simulink model "UNIFIER"  (R2023b)
settings: Solver=ode1  StartTime=0.0  StopTime=60  FixedStep=1/500  RelTol=1e-3
values from neighbouring files (symbols this model uses):
  b = 20.11467    [UNIFIER_LOAD.m]
  c = 1.43676    [UNIFIER_LOAD.m]
  DEP_INTEG_IC = 117.49388    [UNIFIER_LOAD.m]
  Euler0 = [3.43106170068520e-06, 0.0515008506277664, -2.79252663434261]    [UNIFIER_LOAD.m]
  ground_alt = 0    [UNIFIER_LOAD.m]
  h_ref_for_xplane = 0    [UNIFIER_LOAD.m]
  m = 7057    [UNIFIER_LOAD.m]
  omegab0 = [0,0,0]    [UNIFIER_LOAD.m]
  S = 29.98388    [UNIFIER_LOAD.m]
  sensor_delay_steps = 5    [UNIFIER_LOAD.m]
  u1_0 = [2.1112539e-05, -2.1112539e-05, -0.085004635, -0.084972650, 0.19720161, 0.19720161]    [UNIFIER_LOAD.m]
  u2_0 = ones(1,12) .* 0.4252    [UNIFIER_LOAD.m]
  u3_0 = 0.089689    [UNIFIER_LOAD.m]
  u4_0 = 0    [UNIFIER_LOAD.m]
  Vb0 = [52.6789583501891, 0, 2.71559652634250]    [UNIFIER_LOAD.m]
  vtail_dist_to_wing = 7.8070    (= 7.807)    [UNIFIER_LOAD.m]
  vtail_nodes = [dp_VTAIL.Xs_LE;     dp_VTAIL.Ys_LE;     dp_VTAIL.Zs_LE]    [UNIFIER_LOAD.m]
  wing_nodes = [fliplr(dp_WING_tip.LE_Xs),fliplr(dp_WING_root.LE_Xs),dp_WING_root.LE_Xs,dp_WING_tip.LE_Xs;     fliplr(-dp_WING_tip.LE_Ys),fliplr(-dp_WING_root.LE_Ys),dp_WING_root.LE_Ys,dp_WING_tip.LE_Ys;     fliplr(dp_WING_tip.LE_Zs),fliplr(dp_WING_root.LE_Zs),dp_WING_root.LE_Zs,dp_WING_tip.LE_Zs]    [UNIFIER_LOAD.m]
  Xe0 = [0,0,-1100]    [UNIFIER_LOAD.m]
  xyz_cg = [-8.09,0,-0.2]    [UNIFIER_LOAD.m]
  xyz_DEP = [ -6.9629998	-6.9210000	-6.8660002	-6.8099999	-6.7540002	-6.6999998	-6.6999998	-6.7540002	-6.8099999	-6.8660002	-6.9210000	-6.9629998 ... (first row only)    [UNIFIER_LOAD.m]
undefined symbols (not defined in the file or in its folder): dp_DEP, dp_FUSE_FIN, dp_HTU, dp_VTAIL, dp_VTAIL_INDUCED, dp_WING_root, dp_WING_tip, Earth, F, fcc, MIL, WGS84
libraries: aerolibactuator x16, dspnetwork x15, sharedutil x14, simulink_extras x13, sharedtransform x7, aerolibtransform2 x5, simulink x5, aerolibwind2 x4, matrix_library x1, shared6dof x1, aerolibatmos2 x1, slpidlib x1
(part 1 of 4)
settings Model: SimulationMode=rapid-accelerator  PauseTimes=1.5  Creator=johannes  LastModifiedBy=johannes
settings DebuggingCC: ParameterPrecisionLossMsg=none  UnconnectedInputMsg=warning  UnconnectedOutputMsg=warning  UnconnectedLineMsg=warning  UnitsInconsistencyMsg=none  AllowAutomaticUnitConversions=off
settings ModelReferenceCC: EnableRefExpFcnMdlSchedulingChecks=on
settings RTWCC: DLArmComputeVersion=19.05

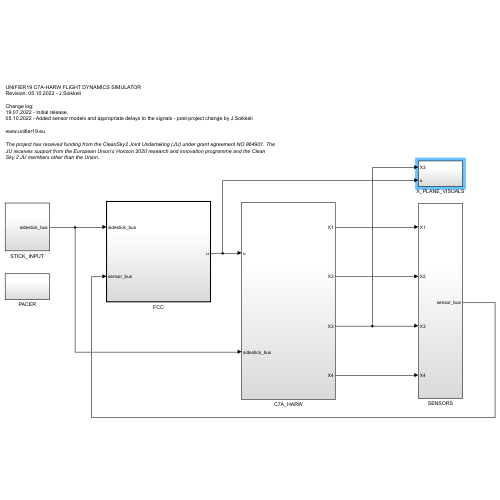
[thumbnail: Simulink's stored preview of the top-level diagram]
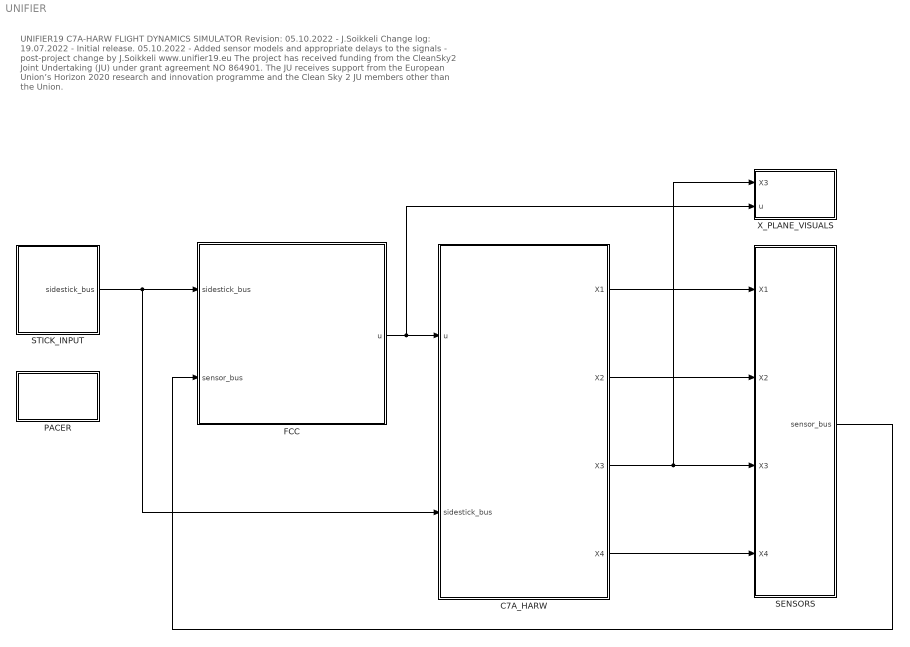
== system UNIFIER ==
  note: UNIFIER19 C7A-HARW FLIGHT DYNAMICS SIMULATOR
      | Revision: 05.10.2022 - J.Soikkeli
      |
      | Change log:
      | 19.07.2022 - Initial release.
      | 05.10.2022 - Added sensor models and appropriate delays to the signals - post-project change by J.Soikkeli
      |
      | www.unifier19.eu
      |
      | The project has received funding from the CleanSky2 Joint Undertaking (JU) under grant agreement NO 864901. The JU receives support from the European Union’s Horizon 2020 research and innovation programme and the Clean Sky 2 JU members other than the Union.
  C7A_HARW : Subsystem
  FCC : Subsystem  TreatAsAtomicUnit=on  SystemSampleTime=fcc.dt
  PACER : Subsystem
  SENSORS : Subsystem
  STICK_INPUT : Subsystem
  X_PLANE_VISUALS : Subsystem
  wires:
  C7A_HARW/3(X3) -> SENSORS/3(X3), X_PLANE_VISUALS/1(X3)
  FCC/1(u) -> X_PLANE_VISUALS/2(u), C7A_HARW/1(u)
  C7A_HARW/1(X1) -> SENSORS/1(X1)
  C7A_HARW/2(X2) -> SENSORS/2(X2)
  C7A_HARW/4(X4) -> SENSORS/4(X4)
  SENSORS/1(sensor_bus) -> FCC/2(sensor_bus)
  STICK_INPUT/1(sidestick_bus) -> C7A_HARW/2(sidestick_bus), FCC/1(sidestick_bus)

== system UNIFIER/C7A_HARW ==
  u : Inport
  sidestick_bus : Inport  Port=2
  Actuator processing and transport delay 10 ms : Delay  DelayLength=5  InitialCondition=repmat([u1_0,u2_0,u3_0,u4_0]',1,5)
  Aero : Subsystem
  Bus Selector : BusSelector  OutputSignals=V_rw_tas,omega_rw,V_rw_mag_tas,beta,alpha,rho
  Cast{1,6..12} (8 alike) : DataTypeConversion  OutDataTypeStr=single  SaturateOnIntegerOverflow=off  RndMeth=Floor
  Demux : Demux  Outputs=[6,12,1,1]
  EOMandEnviroment1 : Subsystem
  FCC frame delay 10 ms (assumed 100Hz FCC) : Delay  DelayLength=5  InitialCondition=repmat([u1_0,u2_0,u3_0,u4_0]',1,5)
  Scopes : Subsystem
  Subsystems : Subsystem
  Sum : Sum  Inputs=|++
  Sum1 : Sum  Inputs=|++
  X1 : Outport
  X2 : Outport  Port=2
  X3 : Outport  Port=3
  X4 : Outport  Port=4
  wires:
  Aero/2(M) -> Sum1/1
  Bus Selector/1 -> Cast7/1  "<V_rw_tas>"
  Bus Selector/6 -> Cast8/1  "<rho>"
  Bus Selector/2 -> Cast9/1  "<omega_rw>"
  Cast6/1 -> Aero/7(DEP_J)
  Subsystems/1(DEP_J) -> Cast6/1
  Subsystems/3(F) -> Sum/2
  Aero/1(F) -> Sum/1
  Sum/1 -> EOMandEnviroment1/1(F)
  Sum1/1 -> EOMandEnviroment1/2(M)
  Subsystems/4(M) -> Sum1/2
  Bus Selector/3 -> Cast10/1  "<V_rw_mag_tas>"
  Bus Selector/4 -> Cast11/1  "<beta>"
  Bus Selector/5 -> Cast12/1  "<alpha>"
  Cast7/1 -> Aero/1(V_rw_tas)
  Cast8/1 -> Aero/6(rho)
  Cast9/1 -> Aero/2(omega_rw)
  Cast10/1 -> Aero/3(V_rw_mag_tas)
  Cast11/1 -> Aero/4(beta)
  Cast12/1 -> Aero/5(alpha)
  Cast1/1 -> Aero/8(u1 (rad))
  Subsystems/2(u1_out (rad)) -> Cast1/1
  EOMandEnviroment1/1(X1) -> Scopes/1(X1), X1/1
  EOMandEnviroment1/4(X4) -> Scopes/4(X4), X4/1, Subsystems/1(X4), Bus Selector/1
  EOMandEnviroment1/2(X2) -> Subsystems/7(X2), X2/1, Scopes/2(X2)
  EOMandEnviroment1/3(X3) -> Subsystems/6(X3), X3/1, Scopes/3(X3)
  Demux/4 -> Aero/9(u4 (gear))
  sidestick_bus/1 -> Subsystems/5(sidestick_bus)
  Demux/3 -> Subsystems/4(u3 (actf))
  Demux/2 -> Subsystems/3(u2 (actf))
  Demux/1 -> Subsystems/2(u1_in (rad))
  u/1 -> FCC frame delay 10 ms (assumed 100Hz FCC)/1
  FCC frame delay 10 ms (assumed 100Hz FCC)/1 -> Actuator processing and transport delay 10 ms/1
  Actuator processing and transport delay 10 ms/1 -> Demux/1

== system UNIFIER/FCC ==
  note: As a part of the UNIFIER19 project, flight control laws (based on non-linear dynamic inversion) were developed. The litearature and findings using these control laws is available on the GIT page.
      |
      | Here we invite you to develop your version of the control laws!
  sidestick_bus : Inport
  sensor_bus : Inport  Port=2
  Bus Selector : BusSelector  OutputSignals=roll_raw,pitch_raw,yaw_raw,throttle_raw
  Constant1 : Constant  Value=u2_0
  Constant2 : Constant  Value=u3_0
  Constant3 : Constant  Value=u1_0
  Constant4 : Constant  SampleTime=-1
  Constant6 : Constant  Value=u4_0
  Manual : Subsystem
  Multiport Switch : MultiPortSwitch  Inputs=2  SaturateOnIntegerOverflow=off  InputSameDT=off
  Mux : Mux
  Terminator : Terminator
  u : Outport
  wires:
  Multiport Switch/1 -> u/1
  Constant3/1 -> Mux/1
  Constant1/1 -> Mux/2
  Constant2/1 -> Mux/3
  Mux/1 -> Multiport Switch/2
  Bus Selector/1 -> Manual/1(aileron)  "<roll_raw>"
  Bus Selector/2 -> Manual/2(elevator)  "<pitch_raw>"
  Bus Selector/3 -> Manual/3(rudder)  "<yaw_raw>"
  Bus Selector/4 -> Manual/4(throttle)  "<throttle_raw>"
  Constant4/1 -> Multiport Switch/1
  Manual/1(u) -> Multiport Switch/3
  Constant6/1 -> Mux/4
  sidestick_bus/1 -> Bus Selector/1
  sensor_bus/1 -> Terminator/1

== system UNIFIER/PACER ==
  note: Soft real time block and associated
      | s-function source codes:
      | - sfun_sleep.c
      | - sfun_getSystemClockTimeval.c
      | - sfun_output_to_console.c
      | are copyrighted
      | by Marc Compere
      | comperem@gmail.com
      | created : 28 May 2018
      | modified: 28 May 2018
  Constant1 : Constant  Value=0
  Constant2 : Constant
  Display : Display
  Manual Switch1 : ManualSwitch  CurrentSetting=0
  Mux : Mux  Inputs=3
  Output to Console : Subsystem  TreatAsAtomicUnit=on
  Subsystem : Subsystem
      settings: OpenFcn=h_fixed=0.001
      mask Display: fprintf('Double-Click to init\nstepsize variable, h_fixed')
  "pace error (s) " : Scope
  simulation time (s)1 : Clock
  soft real time subsystem : Subsystem  mask{t_sample=0.01}
      mask prompts: t_sample "Sleep function interval (s)"
  wires:
  soft real time subsystem/2(pace error (s)) -> "pace error (s) "/1, Display/1, Mux/3
  simulation time (s)1/1 -> Mux/1
  soft real time subsystem/1(t_elapsed_wall_clock (s)) -> Mux/2
  Constant1/1 -> Manual Switch1/2
  Mux/1 -> Output to Console/1(data to console)
  Constant2/1 -> Manual Switch1/1
  Manual Switch1/1 -> Output to Console/Enable

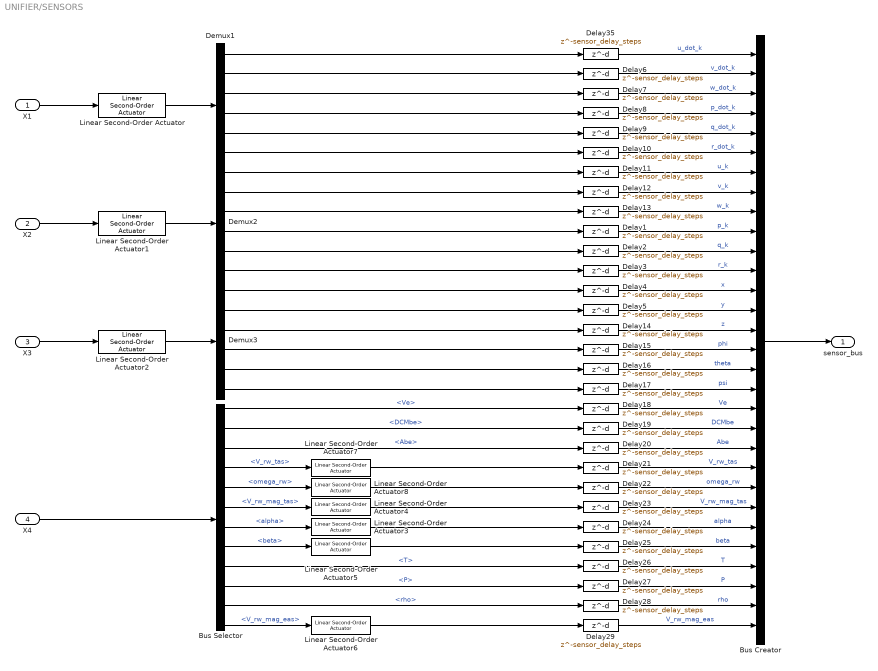
== system UNIFIER/SENSORS ==
  X1 : Inport
  X2 : Inport  Port=2
  X3 : Inport  Port=3
  X4 : Inport  Port=4
  Bus Creator : BusCreator  Inputs=30
  Bus Selector : BusSelector  OutputSignals=Ve,DCMbe,Abe,V_rw_tas,omega_rw,V_rw_mag_tas,alpha,beta,T,P,rho,V_rw_mag_eas
  Delay{1..3,6..10,35} (9 alike) : Delay  DelayLength=sensor_delay_steps
  Delay11 : Delay  DelayLength=sensor_delay_steps  InitialCondition=Vb0(1)
  Delay12 : Delay  DelayLength=sensor_delay_steps  InitialCondition=Vb0(2)
  Delay13 : Delay  DelayLength=sensor_delay_steps  InitialCondition=Vb0(3)
  Delay14 : Delay  DelayLength=sensor_delay_steps  InitialCondition=Xe0(3)
  Delay15 : Delay  DelayLength=sensor_delay_steps  InitialCondition=Euler0(1)
  Delay16 : Delay  DelayLength=sensor_delay_steps  InitialCondition=Euler0(2)
  Delay17 : Delay  DelayLength=sensor_delay_steps  InitialCondition=Euler0(3)
  Delay18 : Delay  DelayLength=sensor_delay_steps  InitialCondition=repmat(Vb0',1,sensor_delay_steps)
  Delay19 : Delay  DelayLength=sensor_delay_steps  InitialCondition=0
  Delay20 : Delay  DelayLength=sensor_delay_steps  InitialCondition=0
  Delay21 : Delay  DelayLength=sensor_delay_steps  InitialCondition=repmat(Vb0',1,sensor_delay_steps)
  Delay22 : Delay  DelayLength=sensor_delay_steps  InitialCondition=0
  Delay23 : Delay  DelayLength=sensor_delay_steps  InitialCondition=sqrt(dot(Vb0,Vb0))
  Delay24 : Delay  DelayLength=sensor_delay_steps  InitialCondition=atan(Vb0(3)/Vb0(1))
  Delay25 : Delay  DelayLength=sensor_delay_steps  InitialCondition=asin(Vb0(2)/sqrt(dot(Vb0,Vb0)))
  Delay26 : Delay  DelayLength=sensor_delay_steps  InitialCondition=273
  Delay27 : Delay  DelayLength=sensor_delay_steps  InitialCondition=101325
  Delay28 : Delay  DelayLength=sensor_delay_steps  InitialCondition=1.225
  Delay29 : Delay  DelayLength=sensor_delay_steps  InitialCondition=sqrt(dot(Vb0,Vb0))
  Delay4 : Delay  DelayLength=sensor_delay_steps  InitialCondition=Xe0(1)
  Delay5 : Delay  DelayLength=sensor_delay_steps  InitialCondition=Xe0(2)
  Demux1 : Demux  Outputs=6
  Demux2 : Demux  Outputs=6
  Demux3 : Demux  Outputs=6
  Linear Second-Order Actuator : aerolibactuator/Linear Second-Order Actuator  wn_fin=30*2*pi  z_fin=1  fin_act_0=zeros(1,6)  fin_act_vel=0
  Linear Second-Order Actuator1 : aerolibactuator/Linear Second-Order Actuator  wn_fin=30*2*pi  z_fin=1  fin_act_0=[Vb0,omegab0]  fin_act_vel=0
  Linear Second-Order Actuator2 : aerolibactuator/Linear Second-Order Actuator  wn_fin=30*2*pi  z_fin=1  fin_act_0=[Xe0,Euler0]  fin_act_vel=0
  Linear Second-Order Actuator3 : aerolibactuator/Linear Second-Order Actuator  wn_fin=5*2*pi  z_fin=1  fin_act_0=atan(Vb0(3)/Vb0(1))  fin_act_vel=0
  Linear Second-Order Actuator4 : aerolibactuator/Linear Second-Order Actuator  wn_fin=5*2*pi  z_fin=1  fin_act_0=sqrt((Vb0(1)^2+Vb0(2)^2+Vb0(3)^2))  fin_act_vel=0
  Linear Second-Order Actuator5 : aerolibactuator/Linear Second-Order Actuator  wn_fin=5*2*pi  z_fin=1  fin_act_0=asin(Vb0(2)/sqrt((Vb0(1)^2+Vb0(2)^2+Vb0(3)^2)))  fin_act_vel=0
  Linear Second-Order Actuator6 : aerolibactuator/Linear Second-Order Actuator  wn_fin=5*2*pi  z_fin=1  fin_act_0=sqrt((Vb0(1)^2+Vb0(2)^2+Vb0(3)^2))  fin_act_vel=0
  Linear Second-Order Actuator7 : aerolibactuator/Linear Second-Order Actuator  wn_fin=5*2*pi  z_fin=1  fin_act_0=Vb0  fin_act_vel=0
  Linear Second-Order Actuator8 : aerolibactuator/Linear Second-Order Actuator  wn_fin=30*2*pi  z_fin=1  fin_act_0=omegab0  fin_act_vel=0
  sensor_bus : Outport
  wires:
  Demux1/1 -> Delay35/1
  Demux1/2 -> Delay6/1
  X4/1 -> Bus Selector/1
  Bus Selector/4 -> Linear Second-Order Actuator7/1  "<V_rw_tas>"
  Bus Selector/5 -> Linear Second-Order Actuator8/1  "<omega_rw>"
  Bus Selector/6 -> Linear Second-Order Actuator4/1  "<V_rw_mag_tas>"
  Bus Selector/7 -> Linear Second-Order Actuator3/1  "<alpha>"
  Bus Selector/8 -> Linear Second-Order Actuator5/1  "<beta>"
  Bus Selector/12 -> Linear Second-Order Actuator6/1  "<V_rw_mag_eas>"
  X1/1 -> Linear Second-Order Actuator/1
  X2/1 -> Linear Second-Order Actuator1/1
  X3/1 -> Linear Second-Order Actuator2/1
  Linear Second-Order Actuator/1 -> Demux1/1
  Linear Second-Order Actuator1/1 -> Demux2/1
  Linear Second-Order Actuator2/1 -> Demux3/1
  Bus Creator/1 -> sensor_bus/1
  Linear Second-Order Actuator6/1 -> Delay29/1
  Bus Selector/11 -> Delay28/1  "<rho>"
  Bus Selector/10 -> Delay27/1  "<P>"
  Bus Selector/9 -> Delay26/1  "<T>"
  Linear Second-Order Actuator5/1 -> Delay25/1
  Linear Second-Order Actuator3/1 -> Delay24/1
  Linear Second-Order Actuator4/1 -> Delay23/1
  Linear Second-Order Actuator8/1 -> Delay22/1
  Linear Second-Order Actuator7/1 -> Delay21/1
  Bus Selector/3 -> Delay20/1  "<Abe>"
  Bus Selector/2 -> Delay19/1  "<DCMbe>"
  Bus Selector/1 -> Delay18/1  "<Ve>"
  Demux3/6 -> Delay17/1
  Demux3/5 -> Delay16/1
  Demux3/4 -> Delay15/1
  Demux3/3 -> Delay14/1
  Demux3/2 -> Delay5/1
  Demux3/1 -> Delay4/1
  Demux2/6 -> Delay3/1
  Demux2/5 -> Delay2/1
  Demux2/4 -> Delay1/1
  Demux2/3 -> Delay13/1
  Demux2/2 -> Delay12/1
  Demux2/1 -> Delay11/1
  Demux1/6 -> Delay10/1
  Demux1/5 -> Delay9/1
  Demux1/4 -> Delay8/1
  Demux1/3 -> Delay7/1
  Delay35/1 -> Bus Creator/1  "u_dot_k"
  Delay6/1 -> Bus Creator/2  "v_dot_k"
  Delay7/1 -> Bus Creator/3  "w_dot_k"
  Delay8/1 -> Bus Creator/4  "p_dot_k"
  Delay9/1 -> Bus Creator/5  "q_dot_k"
  Delay10/1 -> Bus Creator/6  "r_dot_k"
  Delay11/1 -> Bus Creator/7  "u_k"
  Delay12/1 -> Bus Creator/8  "v_k"
  Delay13/1 -> Bus Creator/9  "w_k"
  Delay1/1 -> Bus Creator/10  "p_k"
  Delay2/1 -> Bus Creator/11  "q_k"
  Delay3/1 -> Bus Creator/12  "r_k"
  Delay4/1 -> Bus Creator/13  "x"
  Delay5/1 -> Bus Creator/14  "y"
  Delay14/1 -> Bus Creator/15  "z"
  Delay15/1 -> Bus Creator/16  "phi"
  Delay16/1 -> Bus Creator/17  "theta"
  Delay17/1 -> Bus Creator/18  "psi"
  Delay18/1 -> Bus Creator/19  "Ve"
  Delay19/1 -> Bus Creator/20  "DCMbe"
  Delay20/1 -> Bus Creator/21  "Abe"
  Delay21/1 -> Bus Creator/22  "V_rw_tas"
  Delay22/1 -> Bus Creator/23  "omega_rw"
  Delay23/1 -> Bus Creator/24  "V_rw_mag_tas"
  Delay24/1 -> Bus Creator/25  "alpha"
  Delay25/1 -> Bus Creator/26  "beta"
  Delay26/1 -> Bus Creator/27  "T"
  Delay27/1 -> Bus Creator/28  "P"
  Delay28/1 -> Bus Creator/29  "rho"
  Delay29/1 -> Bus Creator/30  "V_rw_mag_eas"

== system UNIFIER/STICK_INPUT ==
  1-D Lookup Table : Lookup_n-D  NumberOfTableDimensions=1  BreakpointsForDimension1=[0,32770,65540]  IndexSearchMethod=Linear search  BeginIndexSearchUsingPreviousIndexResult=on  Table=[-1,0,1]  ExtrapMethod=Clip  RemoveProtectionInput=on  UseLastTableValue=on  InternalRulePriority=Speed  RndMeth=Simplest
  Bus Creator : BusCreator  Inputs=5
  Constant : Constant  Value=0.5
  Demux : Demux  Outputs=16
  Demux1 : Demux
  Gain : Gain  Gain=0.5
  Mux : Mux  Inputs=12
  Mux1 : Mux
  S-Function : S-Function  FunctionName=sfun_joyinfoex  SFunctionDeploymentMode=off  EnableBusSupport=off
  Sum : Sum  Inputs=++|
  Unary Minus : UnaryMinus
  deviceID : Constant  Value=0
  sidestick_bus : Outport
  wires:
  Demux1/2 -> Bus Creator/2  "pitch_raw"
  Demux1/1 -> Bus Creator/1  "roll_raw"
  Sum/1 -> Bus Creator/3  "throttle_raw"
  Bus Creator/1 -> sidestick_bus/1
  Demux1/4 -> Bus Creator/4  "yaw_raw"
  deviceID/1 -> S-Function/1
  S-Function/1 -> Demux/1
  Demux/5 -> Mux/1
  Demux/6 -> Mux/2
  Demux/7 -> Mux/3
  Demux/8 -> Mux/4
  Demux/9 -> Mux/5
  Demux/10 -> Mux/6
  Demux/11 -> Mux/7
  Demux/12 -> Mux/8
  Demux/13 -> Mux/9
  Demux/14 -> Mux/10
  Demux/15 -> Mux/11
  Demux/16 -> Mux/12
  Mux/1 -> Bus Creator/5  "buttons"
  Demux/1 -> Mux1/1
  Demux/2 -> Mux1/2
  Demux/3 -> Mux1/3
  Demux/4 -> Mux1/4
  Mux1/1 -> 1-D Lookup Table/1
  1-D Lookup Table/1 -> Demux1/1
  Gain/1 -> Sum/2
  Demux1/3 -> Unary Minus/1
  Unary Minus/1 -> Gain/1
  Constant/1 -> Sum/1

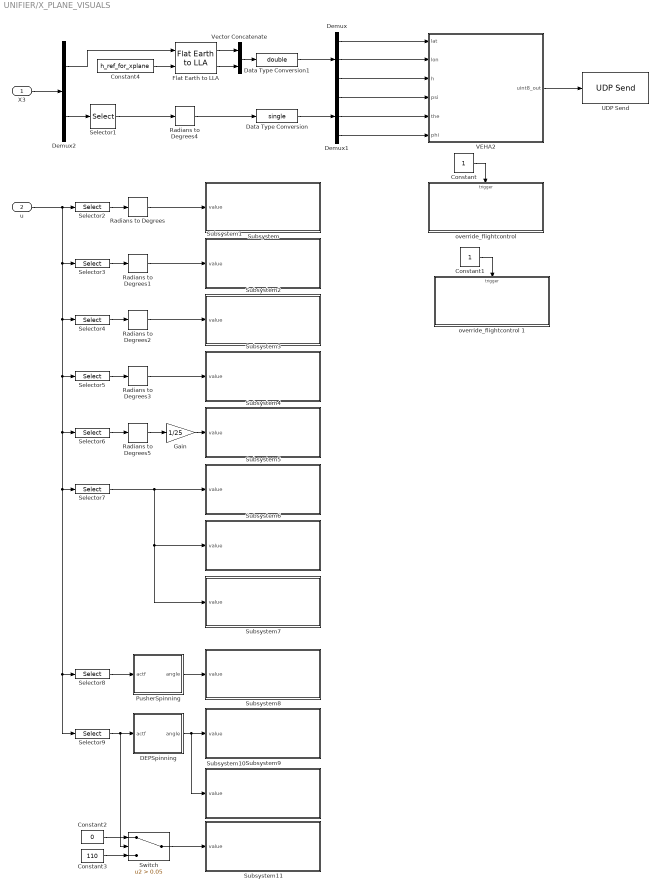
== system UNIFIER/X_PLANE_VISUALS ==
  X3 : Inport
  u : Inport  Port=2
  Constant : Constant
  Constant1 : Constant
  Constant2 : Constant  Value=0
  Constant3 : Constant  Value=110
  Constant4 : Constant  Value=h_ref_for_xplane
  DEPSpinning : Subsystem
  Data Type Conversion : DataTypeConversion  OutDataTypeStr=single  SaturateOnIntegerOverflow=off  RndMeth=Floor
  Data Type Conversion1 : DataTypeConversion  OutDataTypeStr=double  SaturateOnIntegerOverflow=off  RndMeth=Floor
  Demux : Demux  Outputs=3
  Demux1 : Demux  Outputs=3
  Demux2 : Demux  Outputs=2
  Flat Earth to LLA : aerolibtransform2/Flat Earth to LLA  units=Metric (MKS)  ptype=Earth (WGS84)  F=1/298.257223563  R=6378137  refPosPort=off  LL0=latlong0  psi=0
  Gain : Gain  Gain=1/25
  PusherSpinning : Subsystem
  Radians to Degrees{,1..5} (6 alike) : simulink_extras/Transformations/Radians to Degrees
  Selector1 : Selector  InputPortWidth=3  IndexOptions=Index vector (dialog)  Indices=[3,2,1]  OutputSizes=1
  Selector2 : Selector  InputPortWidth=20  IndexOptions=Index vector (dialog)  Indices=1  OutputSizes=1
  Selector3 : Selector  InputPortWidth=20  IndexOptions=Index vector (dialog)  Indices=2  OutputSizes=1
  Selector4 : Selector  InputPortWidth=20  IndexOptions=Index vector (dialog)  Indices=3  OutputSizes=1
  Selector5 : Selector  InputPortWidth=20  IndexOptions=Index vector (dialog)  Indices=4  OutputSizes=1
  Selector6 : Selector  InputPortWidth=20  IndexOptions=Index vector (dialog)  Indices=5  OutputSizes=1
  Selector7 : Selector  InputPortWidth=20  IndexOptions=Index vector (dialog)  Indices=20  OutputSizes=1
  Selector8 : Selector  InputPortWidth=20  IndexOptions=Index vector (dialog)  Indices=19  OutputSizes=1
  Selector9 : Selector  InputPortWidth=20  IndexOptions=Index vector (dialog)  Indices=12  OutputSizes=1
  Subsystem : Subsystem  mask{str='sim/flightmodel/controls/wing1l_ail1def'}
      mask prompts: str "dref"
  Subsystem1 : Subsystem  mask{str='sim/flightmodel/controls/wing1r_ail1def'}
      mask prompts: str "dref"
  Subsystem10 : Subsystem  mask{str='AFormX/Unifier/DEP/PropAngDeg'}
      mask prompts: str "dref"
  Subsystem11 : Subsystem  mask{str='AFormX/Unifier/DEP/DEPAngle'}
      mask prompts: str "dref"
  Subsystem2 : Subsystem  mask{str='sim/flightmodel/controls/mwing02_elv1def'}
      mask prompts: str "dref"
  Subsystem3 : Subsystem  mask{str='sim/flightmodel/controls/mwing01_elv1def'}
      mask prompts: str "dref"
  Subsystem4 : Subsystem  mask{str='sim/flightmodel/controls/flaprat'}
      mask prompts: str "dref"
  Subsystem5 : Subsystem  mask{str='sim/aircraft/parts/acf_gear_deploy[0]'}
      mask prompts: str "dref"
  Subsystem6 : Subsystem  mask{str='sim/aircraft/parts/acf_gear_deploy[1]'}
      mask prompts: str "dref"
  Subsystem7 : Subsystem  mask{str='sim/aircraft/parts/acf_gear_deploy[2]'}
      mask prompts: str "dref"
  Subsystem8 : Subsystem  mask{str='sim/flightmodel2/engines/prop_rotation_angle_deg[0]'}
      mask prompts: str "dref"
  Subsystem9 : Subsystem  mask{str='sim/flightmodel2/engines/prop_rotation_angle_deg[1]'}
      mask prompts: str "dref"
  Switch : Switch  Criteria=u2 > Threshold  Threshold=0.05  SaturateOnIntegerOverflow=off  InputSameDT=off
  UDP Send : dspnetwork/UDP Send  remoteURL='127.0.0.1'  remotePort=49000  localURL='0.0.0.0'  localPortSource=Automatically determine  localPort=-1  sendBufferSize=8192  sampletime=-1  blockPlatform=[]  separateLengthPort=0
  VEHA2 : MATLAB Function  TreatAsAtomicUnit=on
  Vector Concatenate : Concatenate
  "override_flightcontrol " : Subsystem  TreatAsAtomicUnit=on
  override_flightcontrol 1 : Subsystem  TreatAsAtomicUnit=on
  wires:
  Demux/1 -> VEHA2/1(lat)
  Demux/2 -> VEHA2/2(lon)
  Data Type Conversion/1 -> Demux1/1
  Demux1/3 -> VEHA2/6(phi)
  Flat Earth to LLA/1 -> Vector Concatenate/1
  Constant4/1 -> Flat Earth to LLA/2
  VEHA2/1(uint8_out) -> UDP Send/1
  Demux2/2 -> Selector1/1
  Demux1/1 -> VEHA2/4(psi)
  Demux1/2 -> VEHA2/5(the)
  Demux/3 -> VEHA2/3(h)
  Data Type Conversion1/1 -> Demux/1
  Vector Concatenate/1 -> Data Type Conversion1/1
  Flat Earth to LLA/2 -> Vector Concatenate/2
  Demux2/1 -> Flat Earth to LLA/1
  Radians to Degrees4/1 -> Data Type Conversion/1
  Selector1/1 -> Radians to Degrees4/1
  Constant/1 -> "override_flightcontrol "/Trigger
  X3/1 -> Demux2/1
  Selector2/1 -> Radians to Degrees/1
  Radians to Degrees/1 -> Subsystem/1(value)
  Selector3/1 -> Radians to Degrees1/1
  Radians to Degrees1/1 -> Subsystem1/1(value)
  u/1 -> Selector6/1, Selector9/1, Selector8/1, Selector7/1, Selector5/1, Selector4/1, Selector3/1, Selector2/1
  Constant1/1 -> override_flightcontrol 1/Trigger
  Selector4/1 -> Radians to Degrees2/1
  Radians to Degrees2/1 -> Subsystem2/1(value)
  Radians to Degrees3/1 -> Subsystem3/1(value)
  Selector5/1 -> Radians to Degrees3/1
  Radians to Degrees5/1 -> Gain/1
  Gain/1 -> Subsystem4/1(value)
  Selector6/1 -> Radians to Degrees5/1
  Selector7/1 -> Subsystem7/1(value), Subsystem6/1(value), Subsystem5/1(value)
  Selector8/1 -> PusherSpinning/1(actf)
  PusherSpinning/1(angle) -> Subsystem8/1(value)
  DEPSpinning/1(angle) -> Subsystem10/1(value), Subsystem9/1(value)
  Selector9/1 -> Switch/2, DEPSpinning/1(actf)
  Switch/1 -> Subsystem11/1(value)
  Constant2/1 -> Switch/1
  Constant3/1 -> Switch/3

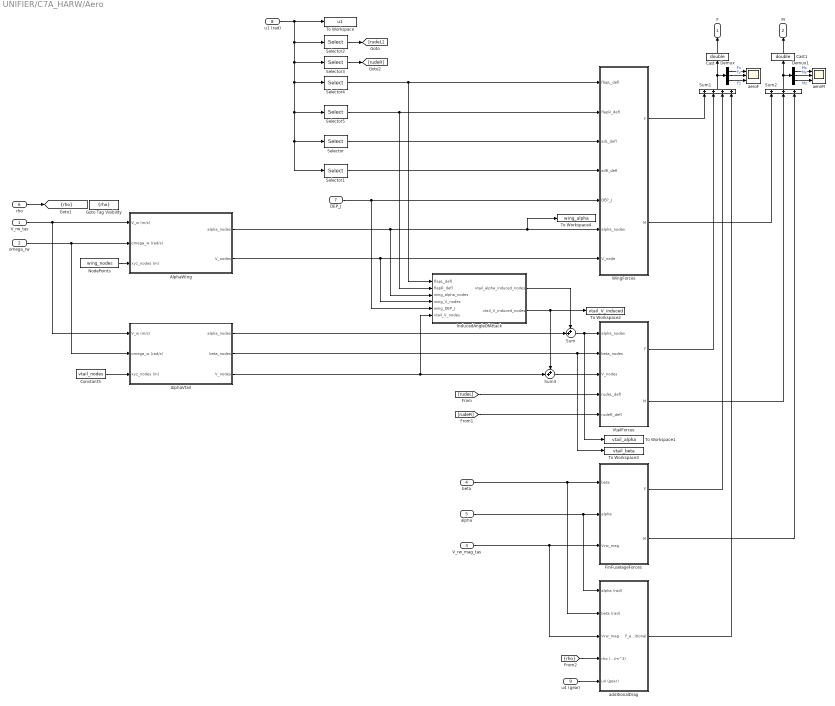
== system UNIFIER/C7A_HARW/Aero ==
  V_rw_tas : Inport  OutDataTypeStr=single  Unit=m/s  PortDimensions=3  LockScale=on
  omega_rw : Inport  Port=2  OutDataTypeStr=single  Unit=rad/s  PortDimensions=3  LockScale=on
  V_rw_mag_tas : Inport  Port=3  OutDataTypeStr=single
  beta : Inport  Port=4  OutDataTypeStr=single
  alpha : Inport  Port=5  OutDataTypeStr=single
  rho : Inport  Port=6  OutDataTypeStr=single  Unit=kg/m^3  PortDimensions=1  LockScale=on
  DEP_J : Inport  Port=7  OutDataTypeStr=single  LockScale=on
  u1 (rad) : Inport  Port=8
  u4 (gear) : Inport  Port=9
  AlphaVtail : Subsystem  TreatAsAtomicUnit=on
  AlphaWIng : Subsystem  TreatAsAtomicUnit=on
  Cast : DataTypeConversion  OutDataTypeStr=double  SaturateOnIntegerOverflow=off  RndMeth=Floor
  Cast1 : DataTypeConversion  OutDataTypeStr=double  SaturateOnIntegerOverflow=off  RndMeth=Floor
  Constant5 : Constant  Value=vtail_nodes
  Demux : Demux  Outputs=3
  Demux1 : Demux  Outputs=3
  FinFuselageForces : Subsystem
  Goto Tag Visibility : GotoTagVisibility  GotoTag=rho
  InducedAngleOfAttack : Subsystem
  NodePoints : Constant  Value=wing_nodes
  Selector : Selector  InputPortWidth=6  IndexOptions=Index vector (dialog)  Indices=1  OutputSizes=1
  Selector1 : Selector  InputPortWidth=6  IndexOptions=Index vector (dialog)  Indices=2  OutputSizes=1
  Selector2 : Selector  InputPortWidth=6  IndexOptions=Index vector (dialog)  Indices=3  OutputSizes=1
  Selector3 : Selector  InputPortWidth=6  IndexOptions=Index vector (dialog)  Indices=4  OutputSizes=1
  Selector4 : Selector  InputPortWidth=6  IndexOptions=Index vector (dialog)  Indices=5  OutputSizes=1
  Selector5 : Selector  InputPortWidth=6  IndexOptions=Index vector (dialog)  Indices=6  OutputSizes=1
  Sum : Sum  Inputs=++|
  Sum1 : Sum  Inputs=++++
  Sum2 : Sum  Inputs=+++
  Sum3 : Sum  Inputs=++|
  To Workspace : ToWorkspace  VariableName=u1  SaveFormat=Structure With Time  SampleTime=1/100
  To Workspace1 : ToWorkspace  VariableName=vtail_alpha  SaveFormat=Structure With Time  SampleTime=1/100
  To Workspace2 : ToWorkspace  VariableName=vtail_V_induced  SaveFormat=Structure With Time  SampleTime=1/100
  To Workspace3 : ToWorkspace  VariableName=vtail_beta  SaveFormat=Structure With Time  SampleTime=1/100
  To Workspace4 : ToWorkspace  VariableName=wing_alpha  SaveFormat=Structure With Time  SampleTime=1/100
  VtailForces : Subsystem
  WingForces : Subsystem
  additionalDrag : Subsystem
  aeroF : Scope  NumInputPorts=3
  aeroM : Scope  NumInputPorts=3
  F : Outport  Unit=N  PortDimensions=3  LockScale=on
  M : Outport  Port=2  Unit=N*m  PortDimensions=3  LockScale=on
  tag scope: rho=scoped
  wires:
  NodePoints/1 -> AlphaWIng/3(xyz_nodes (m))
  Constant5/1 -> AlphaVtail/3(xyz_nodes (m))
  V_rw_tas/1 -> AlphaVtail/1(V_w (m/s)), AlphaWIng/1(V_w (m/s))
  omega_rw/1 -> AlphaVtail/2(omega_w (rad/s)), AlphaWIng/2(omega_w (rad/s))
  AlphaWIng/2(V_nodes) -> WingForces/7(V_node), InducedAngleOfAttack/4(wing_V_nodes)
  DEP_J/1 -> WingForces/5(DEP_J), InducedAngleOfAttack/5(wing_DEP_J)
  Sum/1 -> VtailForces/1(alpha_nodes), To Workspace1/1
  rho/1 -> [rho]
  AlphaVtail/2(beta_nodes) -> VtailForces/2(beta_nodes), To Workspace3/1
  [rudeL] -> VtailForces/4(rudeL_defl)
  [rudeR] -> VtailForces/5(rudeR_defl)
  WingForces/1(F) -> Sum1/1
  VtailForces/1(F) -> Sum1/2
  WingForces/2(M) -> Sum2/1
  VtailForces/2(M) -> Sum2/2
  Sum1/1 -> Demux/1, Cast/1
  AlphaVtail/3(V_nodes) -> InducedAngleOfAttack/6(vtail_V_nodes), Sum3/2
  InducedAngleOfAttack/1(vtail_alpha_induced_nodes) -> Sum/1
  InducedAngleOfAttack/2(vtail_V_induced_nodes) -> To Workspace2/1, Sum3/1
  Sum3/1 -> VtailForces/3(V_nodes)
  AlphaVtail/1(alpha_nodes) -> Sum/2
  Cast/1 -> F/1
  Cast1/1 -> M/1
  V_rw_mag_tas/1 -> FinFuselageForces/3(Vrw_mag), additionalDrag/3(Vrw_mag)
  beta/1 -> FinFuselageForces/1(beta), additionalDrag/2(beta (rad))
  FinFuselageForces/1(F) -> Sum1/3
  FinFuselageForces/2(M) -> Sum2/3
  Selector/1 -> WingForces/3(ailL_defl)
  Selector1/1 -> WingForces/4(ailR_defl)
  Selector4/1 -> WingForces/1(flapL_defl), InducedAngleOfAttack/1(flapL_defl)
  Selector5/1 -> WingForces/2(flapR_defl), InducedAngleOfAttack/2(flapR_defl)
  Selector2/1 -> [rudeL]
  Selector3/1 -> [rudeR]
  Demux/1 -> aeroF/1  "Fx"
  Demux/2 -> aeroF/2  "Fy"
  Demux/3 -> aeroF/3  "Fz"
  Sum2/1 -> Cast1/1, Demux1/1
  Demux1/2 -> aeroM/2  "My"
  Demux1/1 -> aeroM/1  "Mx"
  Demux1/3 -> aeroM/3  "Mz"
  AlphaWIng/1(alpha_nodes) -> WingForces/6(alpha_nodes), To Workspace4/1, InducedAngleOfAttack/3(wing_alpha_nodes)
  alpha/1 -> FinFuselageForces/2(alpha), additionalDrag/1(alpha (rad))
  [rho] -> additionalDrag/4(rho (kg/m^3))
  additionalDrag/1(F_additional) -> Sum1/4
  u4 (gear)/1 -> additionalDrag/5(u4 (gear))
  u1 (rad)/1 -> Selector1/1, Selector/1, Selector5/1, Selector4/1, Selector3/1, Selector2/1, To Workspace/1

== system UNIFIER/C7A_HARW/EOMandEnviroment1 ==
  F : Inport
  M : Inport  Port=2
  Bus Creator : BusCreator  Inputs=12
  Conversion : Subsystem
  EOM: 6DOF (Euler Angles) : shared6dof/6DOF (Euler Angles)  units=Metric (MKS)  mtype=Fixed  rep=Euler Angles  xme_0=Xe0  Vm_0=Vb0  eul_0=Euler0  pm_0=omegab0  mass_0=m  mass_e=0.5  mass_f=2.0  inertia=I  inertia_e=eye(3)  inertia_f=2*eye(3)  k_quat=1.0  vre_flag=on  abi_flag=on  aMode=aMode  xme_statename=''  Vm_statename=''  eul_statename=''  quat_statename=''  pm_statename=''  mass_statename=''
  Enviroment : Subsystem
  Mux : Mux  Inputs=2
  Mux1 : Mux  Inputs=2
  Mux2 : Mux  Inputs=2
  To Workspace : ToWorkspace  VariableName=alpha  SaveFormat=Structure With Time  SampleTime=1/100
  To Workspace1 : ToWorkspace  VariableName=X3  SaveFormat=Structure With Time  SampleTime=1/100
  To Workspace2 : ToWorkspace  VariableName=X2  SaveFormat=Structure With Time  SampleTime=1/100
  To Workspace3 : ToWorkspace  VariableName=X1  SaveFormat=Structure With Time  SampleTime=1/100
  To Workspace4 : ToWorkspace  VariableName=beta  SaveFormat=Structure With Time  SampleTime=1/100
  To Workspace5 : ToWorkspace  VariableName=Vrw_mag  SaveFormat=Structure With Time  SampleTime=1/100
  X1 : Outport
  X2 : Outport  Port=2
  X3 : Outport  Port=3
  X4 : Outport  Port=4
  wires:
  EOM: 6DOF (Euler Angles)/5 -> Enviroment/2(Vb), Mux1/1  "Vb"
  EOM: 6DOF (Euler Angles)/3 -> Mux2/2  "Euler"
  Conversion/3(alpha) -> Bus Creator/7, To Workspace/1  "alpha"
  Mux2/1 -> To Workspace1/1, X3/1
  Enviroment/1(Vrw) -> Bus Creator/4, Conversion/1(Vrw)  "V_rw_tas"
  EOM: 6DOF (Euler Angles)/2 -> Enviroment/1(Xe), Mux2/1  "Xe"
  Enviroment/3(T) -> Bus Creator/9  "T"
  EOM: 6DOF (Euler Angles)/8 -> Mux/1  "Abb"
  Bus Creator/1 -> X4/1
  EOM: 6DOF (Euler Angles)/4 -> Enviroment/3(DCM), Bus Creator/2  "DCMbe"
  EOM: 6DOF (Euler Angles)/6 -> Enviroment/4(omega), Mux1/2  "omegadt"
  Conversion/4(beta) -> To Workspace4/1, Bus Creator/8  "beta"
  Enviroment/5(rho) -> Conversion/2(rho), Bus Creator/11  "rho"
  Conversion/1(Vrw_mag) -> To Workspace5/1, Bus Creator/6  "V_rw_mag_tas"
  EOM: 6DOF (Euler Angles)/7 -> Mux/2  "domegadtdt"
  EOM: 6DOF (Euler Angles)/9 -> Bus Creator/3  "Abe"
  Enviroment/2(omegaw) -> Bus Creator/5  "omega_rw"
  EOM: 6DOF (Euler Angles)/1 -> Bus Creator/1  "Ve"
  Enviroment/4(P) -> Bus Creator/10  "P"
  Mux1/1 -> X2/1, To Workspace2/1
  Mux/1 -> To Workspace3/1, X1/1
  Conversion/2(Vrw_mag_eas) -> Bus Creator/12  "V_rw_mag_eas"
  F/1 -> EOM: 6DOF (Euler Angles)/1
  M/1 -> EOM: 6DOF (Euler Angles)/2

== system UNIFIER/C7A_HARW/Scopes ==
  X1 : Inport
  X2 : Inport  Port=2
  X3 : Inport  Port=3
  X4 : Inport  Port=4
  Bus Selector : BusSelector  OutputSignals=V_rw_mag_tas,V_rw_mag_eas,alpha,beta
  Demux : Demux  Outputs=6
  Demux1 : Demux  Outputs=6
  Demux2 : Demux  Outputs=6
  Radians to Degrees{,1..4} (5 alike) : simulink_extras/Transformations/Radians to Degrees
  Vrw_mag : Scope  NumInputPorts=2
  alphabeta : Scope  NumInputPorts=2
  phithetapsi : Scope  NumInputPorts=3
  pqr : Scope  NumInputPorts=3
  pqr_dot : Scope  NumInputPorts=3
  uvw : Scope  NumInputPorts=3
  uvw_dot : Scope  NumInputPorts=3
  xyz : Scope  NumInputPorts=3
  wires:
  X4/1 -> Bus Selector/1
  Bus Selector/3 -> Radians to Degrees/1  "<alpha>"
  Bus Selector/4 -> Radians to Degrees1/1  "<beta>"
  Bus Selector/1 -> Vrw_mag/1  "<V_rw_mag_tas>"
  Radians to Degrees/1 -> alphabeta/1
  Radians to Degrees1/1 -> alphabeta/2
  X1/1 -> Demux/1
  X2/1 -> Demux1/1
  X3/1 -> Demux2/1
  Demux/1 -> uvw_dot/1
  Demux/2 -> uvw_dot/2
  Demux/3 -> uvw_dot/3
  Demux/4 -> pqr_dot/1
  Demux/5 -> pqr_dot/2
  Demux/6 -> pqr_dot/3
  Bus Selector/2 -> Vrw_mag/2  "<V_rw_mag_eas>"
  Demux1/5 -> pqr/2
  Demux1/6 -> pqr/3
  Demux1/3 -> uvw/3
  Demux1/4 -> pqr/1
  Demux1/2 -> uvw/2
  Demux1/1 -> uvw/1
  Demux2/6 -> Radians to Degrees2/1
  Demux2/1 -> xyz/1
  Demux2/2 -> xyz/2
  Demux2/3 -> xyz/3
  Radians to Degrees2/1 -> phithetapsi/3
  Demux2/5 -> Radians to Degrees4/1
  Radians to Degrees4/1 -> phithetapsi/2
  Demux2/4 -> Radians to Degrees3/1
  Radians to Degrees3/1 -> phithetapsi/1

== system UNIFIER/C7A_HARW/Subsystems ==
  X4 : Inport
  u1_in (rad) : Inport  Port=2
  u2 (actf) : Inport  Port=3
  u3 (actf) : Inport  Port=4
  sidestick_bus : Inport  Port=5
  X3 : Inport  Port=6
  X2 : Inport  Port=7
  Actuators : Subsystem
  DEP : Subsystem
  Gravity : Subsystem
  HTU : Subsystem
  LandingGears : Subsystem
  Scope : Scope
  Scopes : Subsystem
  Sum : Sum  Inputs=++++
  Sum1 : Sum  Inputs=+++
  Sum2 : Sum  Inputs=|++
  DEP_J : Outport
  u1_out (rad) : Outport  Port=2
  F : Outport  Port=3
  M : Outport  Port=4
  wires:
  X2/1 -> LandingGears/1(X2), DEP/1(X2)
  X4/1 -> DEP/2(X4), Gravity/1(X4), HTU/2(X4)
  DEP/1(DEP_J) -> DEP_J/1
  Sum/1 -> F/1
  Gravity/1(F) -> Sum/2
  HTU/1(F (N)) -> Sum/3
  Sum1/1 -> M/1
  HTU/2(M (Nm)) -> Sum1/2
  DEP/2(F) -> Sum/1
  DEP/3(M) -> Sum1/1
  u1_in (rad)/1 -> Scopes/2(cmd), Actuators/1(u1)
  Actuators/1(u1_actual) -> Scopes/1(actual), u1_out (rad)/1
  u3 (actf)/1 -> HTU/1(u3 (actf))
  DEP/4(P (kW)) -> Sum2/1
  HTU/3(P (kW)) -> Sum2/2
  u2 (actf)/1 -> DEP/3(u2 (actf))
  LandingGears/1(F) -> Sum/4
  LandingGears/2(M) -> Sum1/3
  X3/1 -> LandingGears/2(X3)
  sidestick_bus/1 -> LandingGears/3(sidestick_bus)
  Sum2/1 -> Scope/1

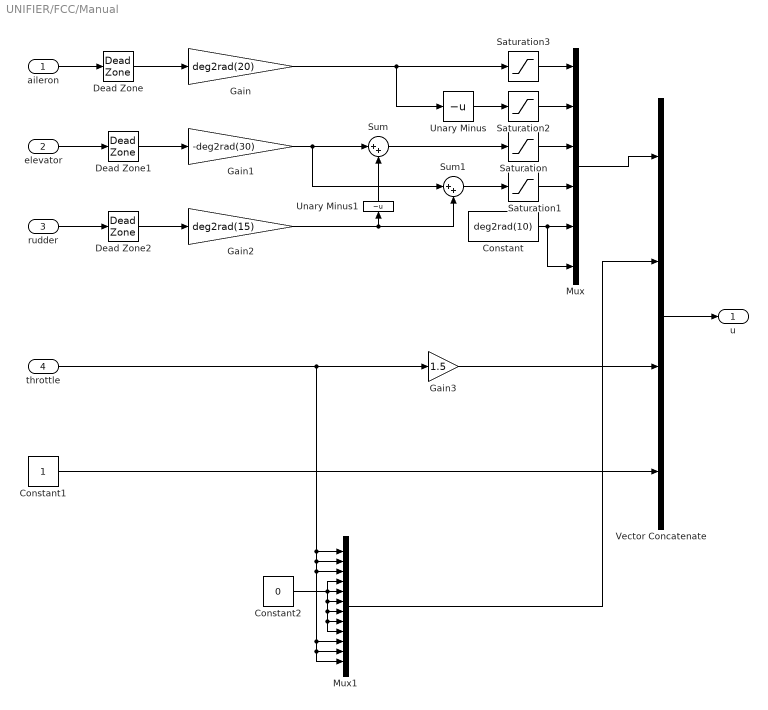
== system UNIFIER/FCC/Manual ==
  aileron : Inport
  elevator : Inport  Port=2
  rudder : Inport  Port=3
  throttle : Inport  Port=4
  Constant : Constant  Value=deg2rad(10)
  Constant1 : Constant
  Constant2 : Constant  Value=0
  Dead Zone : DeadZone  LowerValue=-0.1  UpperValue=0.1
  Dead Zone1 : DeadZone  LowerValue=-0.1  UpperValue=0.1
  Dead Zone2 : DeadZone  LowerValue=-0.1  UpperValue=0.1
  Gain : Gain  Gain=deg2rad(20)
  Gain1 : Gain  Gain=-deg2rad(30)
  Gain2 : Gain  Gain=deg2rad(15)
  Gain3 : Gain  Gain=1.5
  Mux : Mux  Inputs=6
  Mux1 : Mux  Inputs=12
  Saturation : Saturate  UpperLimit=deg2rad(30)  LowerLimit=-deg2rad(30)
  Saturation1 : Saturate  UpperLimit=deg2rad(30)  LowerLimit=-deg2rad(30)
  Saturation2 : Saturate  UpperLimit=deg2rad(20)  LowerLimit=-deg2rad(20)
  Saturation3 : Saturate  UpperLimit=deg2rad(20)  LowerLimit=-deg2rad(20)
  Sum : Sum  Inputs=|++
  Sum1 : Sum  Inputs=|++
  Unary Minus : UnaryMinus
  Unary Minus1 : UnaryMinus
  Vector Concatenate : Concatenate  NumInputs=4
  u : Outport
  wires:
  aileron/1 -> Dead Zone/1
  elevator/1 -> Dead Zone1/1
  Unary Minus/1 -> Saturation2/1
  Gain/1 -> Unary Minus/1, Saturation3/1
  Gain1/1 -> Sum1/1, Sum/1
  Sum1/1 -> Saturation1/1
  Saturation/1 -> Mux/3
  Sum/1 -> Saturation/1
  Saturation1/1 -> Mux/4
  rudder/1 -> Dead Zone2/1
  Gain2/1 -> Sum1/2, Unary Minus1/1
  Saturation2/1 -> Mux/2
  Saturation3/1 -> Mux/1
  Mux/1 -> Vector Concatenate/1
  Vector Concatenate/1 -> u/1
  Constant/1 -> Mux/6, Mux/5
  Mux1/1 -> Vector Concatenate/2
  Unary Minus1/1 -> Sum/2
  Constant1/1 -> Vector Concatenate/4
  Dead Zone/1 -> Gain/1
  Dead Zone1/1 -> Gain1/1
  Dead Zone2/1 -> Gain2/1
  throttle/1 -> Gain3/1, Mux1/1, Mux1/2, Mux1/3, Mux1/12, Mux1/11, Mux1/10
  Constant2/1 -> Mux1/4, Mux1/5, Mux1/9, Mux1/8, Mux1/7, Mux1/6
  Gain3/1 -> Vector Concatenate/3

== system UNIFIER/PACER/Output to Console ==
  note: Note: Constant in green block
      |           can be changed on the fly.
  data to console : Inport
  Enable : EnablePort
  Number of sim steps to skip : Constant  Value=1000
  S-Function : S-Function  FunctionName=sfun_output_to_console  Parameters='[tSimElapsed, tWallElapsed, absTimeErr (s)]: '  SFunctionDeploymentMode=off  EnableBusSupport=off
  skip every N'th : Display
  wires:
  Number of sim steps to skip/1 -> S-Function/1, skip every N'th/1
  data to console/1 -> S-Function/2

== system UNIFIER/PACER/Subsystem ==

== system UNIFIER/PACER/soft real time subsystem ==
  note: What is elapsed real
      | wall-clock time?
  note: What is elapsed
      | simulation time?
  note: Sleep this amount
      | to advance sim time
      | same as wall time
  note: Typically a simple (enough) simulation will fun faster than
      | wall-clock time. This means it's possible for Simulink to
      | simulate, say, 10 seconds in perhps 0.1 or 1 seconds of real
      | wall-clock time.
      |
      | So the challenge is this: how much pause should be inserted
      | every so often to cause the simulation time to advance at
      | the same average rate as real wall-clock time?
      |
      | Using total elapsed time as an absolute reference, this
      | sleep duration will ensure no drift accumulation:
      |
      |      t_sleep = t_elapsed_sim_time - t_elapsed_wall_clock_time
      |
      | Pace error and Sleep() or usleep() resolution is system dependent
      | and likely around 10ms on Windows machines. Better on linux.
      |
      | Marc Compere
      | comperem@gmail.com
      | created : 28 May 2018
      | modified: 29 May 2018
  Constant : Constant  Value=0
  Display : Display
  MinMax : MinMax  Function=max  Inputs=2
  S-Function : S-Function  FunctionName=sfun_sleep  Parameters=t_sample  SFunctionDeploymentMode=off  EnableBusSupport=off
  Sum : Sum  Inputs=|+-
  get elapsed wall-clock time : Subsystem
  s --> ms : Gain  Gain=1000
  simulation time (s) : Clock
  t_elapsed_wall_clock (s) : Outport
  pace error (s) : Outport  Port=2
  wires:
  simulation time (s)/1 -> Sum/1
  Constant/1 -> MinMax/2
  get elapsed wall-clock time/1(t_wall_clock_elapsed (s)) -> t_elapsed_wall_clock (s)/1, Sum/2
  Sum/1 -> Display/1, MinMax/1  "pace error (s)"
  MinMax/1 -> pace error (s)/1, s --> ms/1
  s --> ms/1 -> S-Function/1  "sleep duration (ms)"

== system UNIFIER/X_PLANE_VISUALS/DEPSpinning ==
  note: MAKE THE PUSHER PROP SPIN IN VISUALIZATION
  actf : Inport
  Constant2 : Constant  Value=0
  Constant3 : Constant  Value=10
  Memory1 : Memory  InheritSampleTime=on
  Product : Product
  Scope : Scope
  Sum : Sum  Inputs=|++
  Switch : Switch  Criteria=u2 > Threshold  Threshold=360  SaturateOnIntegerOverflow=off  InputSameDT=off
  angle : Outport
  wires:
  Sum/1 -> Switch/2, Switch/3
  Switch/1 -> angle/1, Memory1/1
  Memory1/1 -> Scope/1, Sum/2
  Product/1 -> Sum/1
  Constant2/1 -> Switch/1
  actf/1 -> Product/1
  Constant3/1 -> Product/2

== system UNIFIER/X_PLANE_VISUALS/PusherSpinning ==
  note: MAKE THE PUSHER PROP SPIN IN VISUALIZATION
  actf : Inport
  Constant2 : Constant  Value=0
  Constant3 : Constant  Value=10
  Memory1 : Memory  InheritSampleTime=on
  Product : Product
  Scope : Scope
  Sum : Sum  Inputs=|++
  Switch : Switch  Criteria=u2 > Threshold  Threshold=360  SaturateOnIntegerOverflow=off  InputSameDT=off
  angle : Outport
  wires:
  Sum/1 -> Switch/2, Switch/3
  Switch/1 -> angle/1, Memory1/1
  Memory1/1 -> Scope/1, Sum/2
  Product/1 -> Sum/1
  Constant2/1 -> Switch/1
  actf/1 -> Product/1
  Constant3/1 -> Product/2

== system UNIFIER/X_PLANE_VISUALS/Subsystem ==
  value : Inport
  Constant : Constant  Value=uint8(str)
  DREF : MATLAB Function  TreatAsAtomicUnit=on
  Data Type Conversion2 : DataTypeConversion  OutDataTypeStr=single  SaturateOnIntegerOverflow=off  RndMeth=Floor
  UDP Send1 : dspnetwork/UDP Send  remoteURL='127.0.0.1'  remotePort=49000  localURL='0.0.0.0'  localPortSource=Automatically determine  localPort=-1  sendBufferSize=8192  sampletime=-1  blockPlatform=[]  separateLengthPort=0
  wires:
  Data Type Conversion2/1 -> DREF/2(value)
  DREF/1(uint8_out) -> UDP Send1/1
  Constant/1 -> DREF/1(str)
  value/1 -> Data Type Conversion2/1

== system UNIFIER/X_PLANE_VISUALS/Subsystem1 ==
  value : Inport
  Constant : Constant  Value=uint8(str)
  DREF : MATLAB Function  TreatAsAtomicUnit=on
  Data Type Conversion2 : DataTypeConversion  OutDataTypeStr=single  SaturateOnIntegerOverflow=off  RndMeth=Floor
  UDP Send1 : dspnetwork/UDP Send  remoteURL='127.0.0.1'  remotePort=49000  localURL='0.0.0.0'  localPortSource=Automatically determine  localPort=-1  sendBufferSize=8192  sampletime=-1  blockPlatform=[]  separateLengthPort=0
  wires:
  Data Type Conversion2/1 -> DREF/2(value)
  DREF/1(uint8_out) -> UDP Send1/1
  Constant/1 -> DREF/1(str)
  value/1 -> Data Type Conversion2/1

== system UNIFIER/X_PLANE_VISUALS/Subsystem10 ==
  value : Inport
  Constant : Constant  Value=uint8(str)
  DREF : MATLAB Function  TreatAsAtomicUnit=on
  Data Type Conversion2 : DataTypeConversion  OutDataTypeStr=single  SaturateOnIntegerOverflow=off  RndMeth=Floor
  UDP Send1 : dspnetwork/UDP Send  remoteURL='127.0.0.1'  remotePort=49000  localURL='0.0.0.0'  localPortSource=Automatically determine  localPort=-1  sendBufferSize=8192  sampletime=-1  blockPlatform=[]  separateLengthPort=0
  wires:
  value/1 -> Data Type Conversion2/1
  Constant/1 -> DREF/1(str)
  DREF/1(uint8_out) -> UDP Send1/1
  Data Type Conversion2/1 -> DREF/2(value)

== system UNIFIER/X_PLANE_VISUALS/Subsystem11 ==
  value : Inport
  Constant : Constant  Value=uint8(str)
  DREF : MATLAB Function  TreatAsAtomicUnit=on
  Data Type Conversion2 : DataTypeConversion  OutDataTypeStr=single  SaturateOnIntegerOverflow=off  RndMeth=Floor
  UDP Send1 : dspnetwork/UDP Send  remoteURL='127.0.0.1'  remotePort=49000  localURL='0.0.0.0'  localPortSource=Automatically determine  localPort=-1  sendBufferSize=8192  sampletime=-1  blockPlatform=[]  separateLengthPort=0
  wires:
  value/1 -> Data Type Conversion2/1
  Constant/1 -> DREF/1(str)
  DREF/1(uint8_out) -> UDP Send1/1
  Data Type Conversion2/1 -> DREF/2(value)

== system UNIFIER/X_PLANE_VISUALS/Subsystem2 ==
  value : Inport
  Constant : Constant  Value=uint8(str)
  DREF : MATLAB Function  TreatAsAtomicUnit=on
  Data Type Conversion2 : DataTypeConversion  OutDataTypeStr=single  SaturateOnIntegerOverflow=off  RndMeth=Floor
  UDP Send1 : dspnetwork/UDP Send  remoteURL='127.0.0.1'  remotePort=49000  localURL='0.0.0.0'  localPortSource=Automatically determine  localPort=-1  sendBufferSize=8192  sampletime=-1  blockPlatform=[]  separateLengthPort=0
  wires:
  value/1 -> Data Type Conversion2/1
  Constant/1 -> DREF/1(str)
  DREF/1(uint8_out) -> UDP Send1/1
  Data Type Conversion2/1 -> DREF/2(value)

== system UNIFIER/X_PLANE_VISUALS/Subsystem3 ==
  value : Inport
  Constant : Constant  Value=uint8(str)
  DREF : MATLAB Function  TreatAsAtomicUnit=on
  Data Type Conversion2 : DataTypeConversion  OutDataTypeStr=single  SaturateOnIntegerOverflow=off  RndMeth=Floor
  UDP Send1 : dspnetwork/UDP Send  remoteURL='127.0.0.1'  remotePort=49000  localURL='0.0.0.0'  localPortSource=Automatically determine  localPort=-1  sendBufferSize=8192  sampletime=-1  blockPlatform=[]  separateLengthPort=0
  wires:
  Data Type Conversion2/1 -> DREF/2(value)
  DREF/1(uint8_out) -> UDP Send1/1
  Constant/1 -> DREF/1(str)
  value/1 -> Data Type Conversion2/1

== system UNIFIER/X_PLANE_VISUALS/Subsystem4 ==
  value : Inport
  Constant : Constant  Value=uint8(str)
  DREF : MATLAB Function  TreatAsAtomicUnit=on
  Data Type Conversion2 : DataTypeConversion  OutDataTypeStr=single  SaturateOnIntegerOverflow=off  RndMeth=Floor
  UDP Send1 : dspnetwork/UDP Send  remoteURL='127.0.0.1'  remotePort=49000  localURL='0.0.0.0'  localPortSource=Automatically determine  localPort=-1  sendBufferSize=8192  sampletime=-1  blockPlatform=[]  separateLengthPort=0
  wires:
  value/1 -> Data Type Conversion2/1
  Constant/1 -> DREF/1(str)
  DREF/1(uint8_out) -> UDP Send1/1
  Data Type Conversion2/1 -> DREF/2(value)

== system UNIFIER/X_PLANE_VISUALS/Subsystem5 ==
  value : Inport
  Constant : Constant  Value=uint8(str)
  DREF : MATLAB Function  TreatAsAtomicUnit=on
  Data Type Conversion2 : DataTypeConversion  OutDataTypeStr=single  SaturateOnIntegerOverflow=off  RndMeth=Floor
  UDP Send1 : dspnetwork/UDP Send  remoteURL='127.0.0.1'  remotePort=49000  localURL='0.0.0.0'  localPortSource=Automatically determine  localPort=-1  sendBufferSize=8192  sampletime=-1  blockPlatform=[]  separateLengthPort=0
  wires:
  value/1 -> Data Type Conversion2/1
  Constant/1 -> DREF/1(str)
  DREF/1(uint8_out) -> UDP Send1/1
  Data Type Conversion2/1 -> DREF/2(value)

== system UNIFIER/X_PLANE_VISUALS/Subsystem6 ==
  value : Inport
  Constant : Constant  Value=uint8(str)
  DREF : MATLAB Function  TreatAsAtomicUnit=on
  Data Type Conversion2 : DataTypeConversion  OutDataTypeStr=single  SaturateOnIntegerOverflow=off  RndMeth=Floor
  UDP Send1 : dspnetwork/UDP Send  remoteURL='127.0.0.1'  remotePort=49000  localURL='0.0.0.0'  localPortSource=Automatically determine  localPort=-1  sendBufferSize=8192  sampletime=-1  blockPlatform=[]  separateLengthPort=0
  wires:
  value/1 -> Data Type Conversion2/1
  Constant/1 -> DREF/1(str)
  DREF/1(uint8_out) -> UDP Send1/1
  Data Type Conversion2/1 -> DREF/2(value)

== system UNIFIER/X_PLANE_VISUALS/Subsystem7 ==
  value : Inport
  Constant : Constant  Value=uint8(str)
  DREF : MATLAB Function  TreatAsAtomicUnit=on
  Data Type Conversion2 : DataTypeConversion  OutDataTypeStr=single  SaturateOnIntegerOverflow=off  RndMeth=Floor
  UDP Send1 : dspnetwork/UDP Send  remoteURL='127.0.0.1'  remotePort=49000  localURL='0.0.0.0'  localPortSource=Automatically determine  localPort=-1  sendBufferSize=8192  sampletime=-1  blockPlatform=[]  separateLengthPort=0
  wires:
  value/1 -> Data Type Conversion2/1
  Constant/1 -> DREF/1(str)
  DREF/1(uint8_out) -> UDP Send1/1
  Data Type Conversion2/1 -> DREF/2(value)

== system UNIFIER/X_PLANE_VISUALS/Subsystem8 ==
  value : Inport
  Constant : Constant  Value=uint8(str)
  DREF : MATLAB Function  TreatAsAtomicUnit=on
  Data Type Conversion2 : DataTypeConversion  OutDataTypeStr=single  SaturateOnIntegerOverflow=off  RndMeth=Floor
  UDP Send1 : dspnetwork/UDP Send  remoteURL='127.0.0.1'  remotePort=49000  localURL='0.0.0.0'  localPortSource=Automatically determine  localPort=-1  sendBufferSize=8192  sampletime=-1  blockPlatform=[]  separateLengthPort=0
  wires:
  value/1 -> Data Type Conversion2/1
  Constant/1 -> DREF/1(str)
  DREF/1(uint8_out) -> UDP Send1/1
  Data Type Conversion2/1 -> DREF/2(value)

== system UNIFIER/X_PLANE_VISUALS/Subsystem9 ==
  value : Inport
  Constant : Constant  Value=uint8(str)
  DREF : MATLAB Function  TreatAsAtomicUnit=on
  Data Type Conversion2 : DataTypeConversion  OutDataTypeStr=single  SaturateOnIntegerOverflow=off  RndMeth=Floor
  UDP Send1 : dspnetwork/UDP Send  remoteURL='127.0.0.1'  remotePort=49000  localURL='0.0.0.0'  localPortSource=Automatically determine  localPort=-1  sendBufferSize=8192  sampletime=-1  blockPlatform=[]  separateLengthPort=0
  wires:
  value/1 -> Data Type Conversion2/1
  Constant/1 -> DREF/1(str)
  DREF/1(uint8_out) -> UDP Send1/1
  Data Type Conversion2/1 -> DREF/2(value)

== system UNIFIER/X_PLANE_VISUALS/override_flightcontrol  ==
  Trigger : TriggerPort  VariantControl=(inherit)  InitialTriggerSignalState=zero
  Constant : Constant
  Subsystem : Subsystem  mask{str='sim/operation/override/override_flightcontrol'}
      mask prompts: str "dref"
  wires:
  Constant/1 -> Subsystem/1(value)

== system UNIFIER/X_PLANE_VISUALS/override_flightcontrol 1 ==
  Trigger : TriggerPort  VariantControl=(inherit)  InitialTriggerSignalState=zero
  Constant : Constant
  Subsystem : Subsystem  mask{str='sim/operation/override/override_control_surfaces'}
      mask prompts: str "dref"
  wires:
  Constant/1 -> Subsystem/1(value)

== system UNIFIER/C7A_HARW/Aero/AlphaVtail ==
  V_w (m/s) : Inport
  omega_w (rad/s) : Inport  Port=2
  xyz_nodes (m) : Inport  Port=3  Partition=on  PartitionDimension=2  PartitionWidth=1  PartitionOffset=0
  3x3 Cross Product : sharedutil/3x3 Cross Product  aMode=aMode
  Asin : Trigonometry  Operator=asin
  Atan : Trigonometry  Operator=atan
  Cast : DataTypeConversion  OutDataTypeStr=single  SaturateOnIntegerOverflow=off  RndMeth=Floor
  Constant : Constant  Value=xyz_cg
  Constant1 : Constant  Value=eps  OutDataTypeStr=single
  Demux : Demux  Outputs=3
  Divide : Product  Inputs=*/
  Divide1 : Product  Inputs=*/
  For Each : ForEach  DisableCoverage=on  SpecifiedNumIters=16
  Mux : Mux  Inputs=3
  Sum : Sum  Inputs=+-
  Sum1 : Sum  Inputs=++|
  Sum2 : Sum  Inputs=|++
  Sum3 : Sum  Inputs=|++
  V_inf : Fcn  Expr=sqrt(u(1)^2+u(2)^2+u(3)^2)
  alpha_nodes : Outport  ConcatenationDimension=2
  beta_nodes : Outport  Port=2  ConcatenationDimension=2
  V_nodes : Outport  Port=3  ConcatenationDimension=2
  wires:
  3x3 Cross Product/1 -> Sum1/1
  Sum/1 -> 3x3 Cross Product/1
  Constant/1 -> Cast/1
  xyz_nodes (m)/1 -> Sum/2
  omega_w (rad/s)/1 -> 3x3 Cross Product/2
  V_w (m/s)/1 -> Sum1/2
  Sum1/1 -> Demux/1
  Demux/1 -> Sum2/1, Mux/1  "u"
  Demux/3 -> Mux/3, Divide/1  "w"
  Divide/1 -> Atan/1
  Atan/1 -> alpha_nodes/1
  Sum2/1 -> Divide/2
  Constant1/1 -> Sum3/2, Sum2/2
  Divide1/1 -> Asin/1
  Demux/2 -> Mux/2, Divide1/1
  Mux/1 -> V_inf/1
  Asin/1 -> beta_nodes/1  "beta"
  V_inf/1 -> Sum3/1
  Sum3/1 -> V_nodes/1, Divide1/2
  Cast/1 -> Sum/1

== system UNIFIER/C7A_HARW/Aero/AlphaWIng ==
  V_w (m/s) : Inport
  omega_w (rad/s) : Inport  Port=2
  xyz_nodes (m) : Inport  Port=3  Partition=on  PartitionDimension=2  PartitionWidth=1  PartitionOffset=0
  Cast : DataTypeConversion  OutDataTypeStr=single  SaturateOnIntegerOverflow=off  RndMeth=Floor
  ComputeAlphaBetaV : Subsystem
  Constant : Constant  Value=xyz_cg
  Cross Product : matrix_library/Cross Product
  For Each : ForEach  DisableCoverage=on  SpecifiedNumIters=14
  Sum : Sum  Inputs=+-
  Sum1 : Sum  Inputs=++|
  Terminator : Terminator
  alpha_nodes : Outport  ConcatenationDimension=2
  V_nodes : Outport  Port=2  ConcatenationDimension=2
  wires:
  Cross Product/1 -> Sum1/1
  Sum/1 -> Cross Product/1
  Constant/1 -> Cast/1
  xyz_nodes (m)/1 -> Sum/2
  omega_w (rad/s)/1 -> Cross Product/2
  V_w (m/s)/1 -> Sum1/2
  Cast/1 -> Sum/1
  Sum1/1 -> ComputeAlphaBetaV/1(V_w_local)
  ComputeAlphaBetaV/3(V_nodes) -> V_nodes/1
  ComputeAlphaBetaV/2(beta_nodes) -> Terminator/1
  ComputeAlphaBetaV/1(alpha_nodes) -> alpha_nodes/1
